simulink model "import_graph_sol"  (R2020a)
settings: Solver=VariableStepAuto  StartTime=0.0  StopTime=32*128 - 1  RelTol=1e-3
InitFcn:
  | xmcCheckSlxPath(bdroot);
  | input = readcomplexdata('input.txt');
  | assignin('base', 'input', input);
undefined symbols (not defined in the file or in its folder): GraphClass, namespace, xc7vx485tffg1157
libraries: ModelComposer x2, dspsrcs4 x1
settings Model: Creator=viswanad  LastModifiedBy=viswanad
settings DataIOCC: ReturnWorkspaceOutputs=off
settings SFSimCC: CustomCodeUndefinedFunction=UseInterfaceOnly

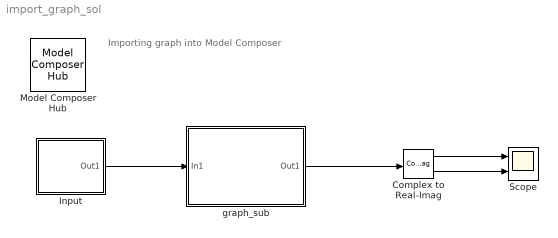
== system import_graph_sol ==
  note: Importing graph into Model Composer
  Complex to Real-Imag : ComplexToRealImag
  Input : Subsystem
  Model Composer Hub : ModelComposer/Model Composer Hub  CodeGeneration=off  SubsystemName=graph_sub  TargetDirectory=./code  ExportType=AI Engines  IpVendor=xilinx.com  IpLibrary=hls  IpVersion=1.0  IpHWLanguage=Verilog  AieCompilerOptions={}  CreateTestbench=on  TestbenchStackSize=10  RunAieSim=off  AieSimTimeout=1500000  RunAieSimProfiling=off  LaunchVitisAnalyzer=off  PlotOutput=off  RunX86Sim=on  X86SimTimeout=10  GenHwImage=off  PlatformType=Not Specified  ProjDevice=xc7vx485tffg1157-1  ProjDevicePart=xc7vx485tffg1157-1  SamplePeriod=-1  ClockFrequency=200  DataPathParallelism=1
  Scope : Scope  NumInputPorts=2
  graph_sub : Subsystem
  wires:
  Complex to Real-Imag/2 -> Scope/2
  Complex to Real-Imag/1 -> Scope/1
  graph_sub/1(Out1) -> Complex to Real-Imag/1
  Input/1(Out1) -> graph_sub/1(In1)

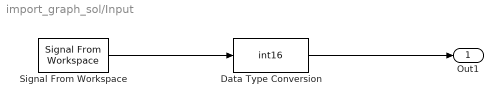
== system import_graph_sol/Input ==
  Data Type Conversion : DataTypeConversion  OutDataTypeStr=int16
  Signal From Workspace : dspsrcs4/Signal From Workspace  X=input  Ts=1  nsamps=128  OutputAfterFinalValue=Setting to zero  ignoreOrWarnInputAndFrameLengths=off  OutputFrames=off
  Out1 : Outport  VectorParamsAs1DForOutWhenUnconnected=off
  wires:
  Signal From Workspace/1 -> Data Type Conversion/1
  Data Type Conversion/1 -> Out1/1

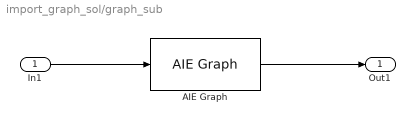
== system import_graph_sol/graph_sub ==
  In1 : Inport
  AIE Graph : ModelComposer/AIE Graph  PortAttributesTable={'Input', 'In1', 'window', 'cint16', '128', 'sync', '';'Output', 'Out1', 'window', 'cint16', '128', 'sync', ''}  PortAttributesEnablement={'off', 'on', 'off', 'off', 'off', 'off', 'off';'off', 'on', 'off', 'off', 'off', 'off', 'off'}  SampleTime=-1  ClassDeclTypeOptions=C[1 1]@t7@<empty>  ClassDecl=<empty>  ClassTemplateParams={}  ClassTemplateParamsEnables={}  ClassPortParams={}  ClassCtorDeclTypeOptions=C[1 1]@t7@<empty>  ClassCtorDecl=<empty>  ClassCtorParams={}  PortArgDecls={'in window cint16 in1'; 'out window cint16 out1'}  PortGraphPortNames={'In1'; 'Out1'}  PortTypes={'window'; 'window'}  PortDataTypes={'cint16'; 'cint16'}  PortSizes={1.280000000000000000e+02; 1.280000000000000000e+02}  PortSynchronicities={'sync'; 'sync'}  PortSignalSizes={0.000000000000000000e+00, 0.000000000000000000e+00}  SimLibPath=''  ClassIndex=0  ClassCtorIndex=0  ClassTabVisible=off  FunctionTabVisible=on  GraphFileSelect=Source file (*.cpp)  GraphClassName=namespace::GraphClass  GraphName=Aie_system  GraphHeaderFiles={'aie_system.h'}  GraphSourceFile=aie_system.cpp  GraphSearchPaths={'./kernels/src', './kernels/inc', './include'}  GraphPreProcOptions={}  blockJsonConstraints=[]  deprecateConstraints=0
  Out1 : Outport  VectorParamsAs1DForOutWhenUnconnected=off
  wires:
  In1/1 -> AIE Graph/1
  AIE Graph/1 -> Out1/1
